simulink model "AZ12"  (R2020a)
settings: Solver=VariableStepAuto  StartTime=0.0  StopTime=6  RelTol=1e-3
libraries: fl_lib x109, ee_lib x35, nesl_utility x16, simulink x3, fl_ps_legacy_lib x1
(part 1 of 2)
settings Model: Creator=sakht system  LastModifiedBy=sakht system

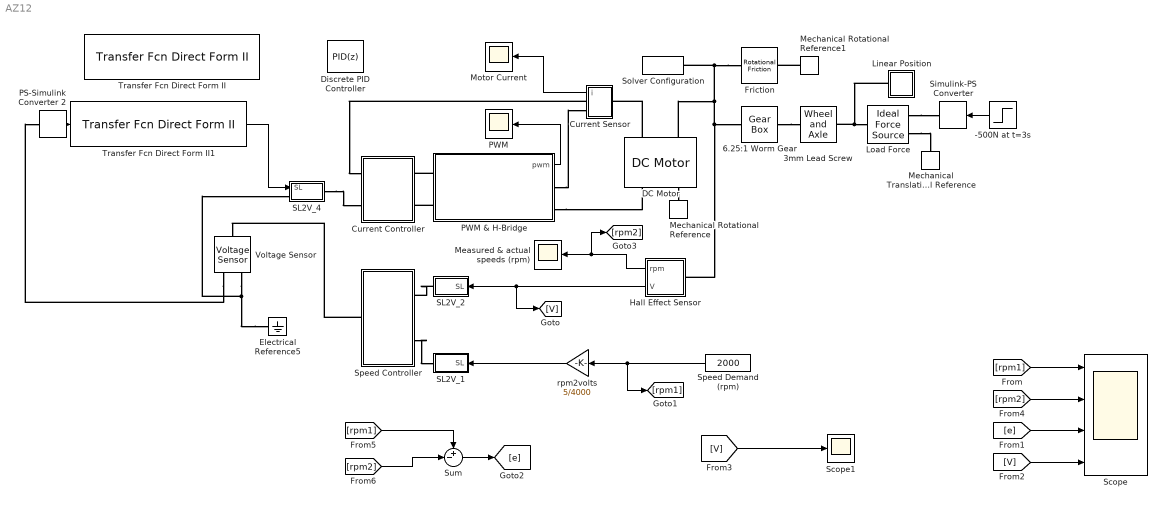
== system AZ12 ==
  -500N at t=3s : Step  Time=3  After=0  SampleTime=0
  3mm Lead Screw : fl_lib/Mechanical/Mechanisms/Wheel and Axle  R=3e-3/(2*pi) m  or=1  t_specify=off  t_priority=High  t=0 N*m  t_nominal_specify=off  t_nominal_unit=N*m  t_nominal_value=1  f_specify=off  f_priority=High  f=0 N  f_nominal_specify=off  f_nominal_unit=N  f_nominal_value=1
  6.25:1 Worm Gear : fl_lib/Mechanical/Mechanisms/Gear Box  ratio=6.25  t_in_specify=off  t_in_priority=High  t_in=0 N*m  t_in_nominal_specify=off  t_in_nominal_unit=N*m  t_in_nominal_value=1  t_out_specify=off  t_out_priority=High  t_out=0 N*m  t_out_nominal_specify=off  t_out_nominal_unit=N*m  t_out_nominal_value=1
  Current Controller : Subsystem
  Current Sensor : Subsystem
  DC Motor : ee_lib/Electromechanical/Brushed Motors/DC Motor  field_option=ee.enum.field_option.pm  Rf=100 Ohm  Lf=1 H  Laf=0.15 H  If0=0 A  parameterization=1  Ra=4.8 Ohm  La=1600e-6 H  emf_or_torque=2  Kv=0.0637 V/rpm  Ki=0.066 N*m/A  T_stall=3e-3*4000/(2*pi*6.25) N*m  w_max=3250 rpm  w_rated=2375 rpm  P_rated=19 W  V_rated=24 V  J=2.5e-5 kg*m^2  lam_param=1  lam=1e-08 N*m/(rad/s)  i_noload=0 A  V_i_noload=1.5 V  speed0=0 rpm  alpha=3.93e-3 1/K  Tmeas=25 degC  thermal_mass=100 J/K  initial_temperature=25 degC
  Discrete PID Controller : simulink/Continuous/PID Controller  Controller=PID  Form=Parallel  TimeDomain=Discrete-time  UseExternalTs=off  SampleTime=0.002  IntegratorMethod=Forward Euler  FilterMethod=Forward Euler  ControllerParametersSource=internal  P=2.4  I=5  D=0.02  UseFilter=on  N=10  TunerSelectOption=Transfer Function Based (PID Tuner App)  InitialConditionSource=internal  InitialConditionForIntegrator=0  InitialConditionForFilter=0  DifferentiatorICPrevScaledInput=0  ExternalReset=none  TrackingMode=off  Kt=1  LimitOutput=off  UpperSaturationLimit=inf  LowerSaturationLimit=-inf  LinearizeAsGain=off  AntiWindupMode=none  Kb=1  POutMin=[]  POutMax=[]  IOutMin=[]  IOutMax=[]  DOutMin=[]  DOutMax=[]  NOutMin=[]  NOutMax=[]  SumOutMin=[]  SumOutMax=[]  SaturationOutMin=[]  SaturationOutMax=[]  PParamMin=[]  PParamMax=[]  IParamMin=[]  IParamMax=[]  DParamMin=[]  DParamMax=[]  NParamMin=[]  NParamMax=[]  KbParamMin=[]  KbParamMax=[]  KtParamMin=[]  KtParamMax=[]  KbOutMin=[]  KbOutMax=[]  KtOutMin=[]  KtOutMax=[]  IntegratorOutMin=[]  IntegratorOutMax=[]  FilterOutMin=[]  FilterOutMax=[]  SumI1OutMin=[]  SumI1OutMax=[]  SumI2OutMin=[]  SumI2OutMax=[]  SumI3OutMin=[]  SumI3OutMax=[]  SumI4OutMin=[]  SumI4OutMax=[]  SumDOutMin=[]  SumDOutMax=[]  DifferentiatorOutMin=[]  DifferentiatorOutMax=[]  FilterDiffOutCoefMin=[]  FilterDiffOutCoefMax=[]  ReciprocalOutMin=[]  ReciprocalOutMax=[]  SumDenOutMin=[]  SumDenOutMax=[]  SumNumOutMin=[]  SumNumOutMax=[]  DivideOutMin=[]  DivideOutMax=[]  UdiffTsProdOutMin=[]  UdiffTsProdOutMax=[]  NTsProdOutMin=[]  NTsProdOutMax=[]  UintegralTsProdOutMin=[]  UintegralTsProdOutMax=[]  UngainTsProdOutMin=[]  UngainTsProdOutMax=[]  IntegratorContinuousStateAttributes=''  IntegratorStateMustResolveToSignalObject=off  IntegratorRTWStateStorageClass=Auto  FilterContinuousStateAttributes=''  FilterStateMustResolveToSignalObject=off  FilterRTWStateStorageClass=Auto  ParallelPVariant=InternalParameters  IdealPVariant=Disabled  IVariant=InternalParameters  DVariant=InternalParameters  IntegratorVariant=Discrete  SatVariant=Disabled  AWVariant=Passthrough  PCopyVariant=Disabled  TRVariant=Disabled  FdbkBlocksVariant=Forward  IdealPFdbkVariant=Disabled  SatFdbkVariant=Disabled  DerivativeFilterVariant=ForwardEulerFilter  NVariant=InternalParameters  NCopyVariant=Disabled  FilterICVariant=InternalICsFilter  IntegratorICVariant=InternalICs  ExternalResetVariant=Disabled  TRSumVariant=Passthrough  SumFdbkVariant=Disabled  SumVariant=Sum_PID  TsampFilterVariant=InternalTs  TsampNgainVariant=Passthrough  TsampIntegralVariant=Passthrough
  Electrical Reference5 : fl_lib/Electrical/Electrical Elements/Electrical Reference
  Friction : fl_lib/Mechanical/Rotational Elements/Rotational Friction  brkwy_trq=0.022 N*m  brkwy_vel=0.03347 rad/s  Col_trq=0.022 N*m  visc_coef=0 N*m/(rad/s)  w_specify=off  w_priority=High  w=0 rad/s  w_nominal_specify=off  w_nominal_unit=rad/s  w_nominal_value=1  t_specify=off  t_priority=High  t=0 N*m  t_nominal_specify=off  t_nominal_unit=N*m  t_nominal_value=1
  Hall Effect Sensor : Subsystem
  Linear Position : Subsystem
  Load Force : fl_lib/Mechanical/Mechanical Sources/Ideal Force Source
  Measured & actual speeds (rpm) : Scope
  Mechanical Rotational Reference : fl_lib/Mechanical/Rotational Elements/Mechanical Rotational Reference
  Mechanical Rotational Reference1 : fl_lib/Mechanical/Rotational Elements/Mechanical Rotational Reference
  Mechanical Translational Reference : fl_lib/Mechanical/Translational Elements/Mechanical Translational Reference
  Motor Current : Scope
  PS-Simulink Converter 2 : nesl_utility/PS-Simulink Converter  PhysicalDomain=network_engine_domain  SubClassName=ps_output  LeftPortType=input  RightPortType=output  PseudoPeriodic=off  Frequencies=[]  Unit=V  AffineConversion=off
  PWM : Scope
  PWM & H-Bridge : Subsystem  Variant=on  VariantControlMode=Label  LabelModeActiveChoice=pwm_choice==1
      settings: AttributesFormatString=%<BlockChoice>
  SL2V_1 : Subsystem
  SL2V_2 : Subsystem
  SL2V_4 : Subsystem
  Scope : Scope  NumInputPorts=4
  Scope1 : Scope
  Simulink-PS Converter : nesl_utility/Simulink-PS Converter  PhysicalDomain=network_engine_domain  SubClassName=ps_input  LeftPortType=input  RightPortType=output  PseudoPeriodic=off  Frequencies=[]  NoiseDistribution=none  NoiseParameters=[]  Unit=N  AffineConversion=off  FilteringAndDerivatives=zero  SimscapeFilterOrder=1  InputFilterTimeConstant=.001  UdotUserProvided=0
  Solver Configuration : nesl_utility/Solver Configuration  PhysicalDomain=network_engine_domain  SubClassName=solver  LeftPortType=input  RightPortType=generic  Tones=[]  Harmonics=[]  SimulateNoise=off  Profile=off  UseLocalSampling=off  EnableSwitchedLinearOptims=on  FrequencyDomain=off  UseCCode=off  RelTol=0.001  AbsTol=1e-06  MinStep=1e-09  ToWorkspace=off  RevertToSquareIcSolve=off  NumHomotopyIterations=100  PhasorMode=off  PhasorModeNumHarmonics=1  DoDC=off  ResidualTolerance=1e-9  UseLocalSolver=off  LocalSolverChoice=NE_BACKWARD_EULER_ADVANCER  LocalSolverSampleTime=.001  DoFixedCost=off  MaxNonlinIter=3  MaxModeIter=2  LinearAlgebra=Sparse  EquationFormulation=NE_TIME_EF  DelaysMemoryBudget=1024  AutomaticFiltering=on  FilteringTimeConstant=0.001  PartitionStorageMethod=AS_NEEDED  PartitionMemoryBudget=1024  PartitionMethod=FAST
  Speed Controller : Subsystem
  Speed Demand (rpm) : Constant  Value=2000
  Sum : Sum  Inputs=+-|
  Transfer Fcn Direct Form II : simulink/Additional Math & Discrete/Additional Discrete/Transfer Fcn Direct Form II  NumCoefVec=[0.31 -0.0034 0]  DenCoefVec=[-0.0058 0]  vinit=0.0  DoSatur=off
      settings: SourceProductBaseCode=SL
  Transfer Fcn Direct Form II1 : simulink/Additional Math & Discrete/Additional Discrete/Transfer Fcn Direct Form II  NumCoefVec=[0.017 -0.0044 0.00340]  DenCoefVec=[0 -0.00077 -0.002]  vinit=0.0  DoSatur=off
      settings: SourceProductBaseCode=SL
  Voltage Sensor : fl_lib/Electrical/Electrical Sensors/Voltage Sensor
  rpm2volts : Gain  Gain=5/4000
  wires:
  [V] -> Scope/4
  [rpm1] -> Scope/1
  Hall Effect Sensor/1(rpm) -> [rpm2], Measured & actual speeds (rpm)/1
  [V] -> Scope1/1
  [rpm2] -> Scope/2
  rpm2volts/1 -> SL2V_1/1(SL)
  [e] -> Scope/3
  Current Sensor/1(i) -> Motor Current/1
  Speed Demand (rpm)/1 -> rpm2volts/1, [rpm1]
  -500N at t=3s/1 -> Simulink-PS Converter/1
  Transfer Fcn Direct Form II1/1 -> SL2V_4/1(SL)
  Hall Effect Sensor/2(V) -> [V], SL2V_2/1(SL)
  PWM & H-Bridge/1(pwm) -> PWM/1
  PS-Simulink Converter 2/1 -> Transfer Fcn Direct Form II1/1
  Sum/1 -> [e]
  [rpm1] -> Sum/1
  [rpm2] -> Sum/2
  connections:
  Friction/LConn1 -- Hall Effect Sensor/LConn1 -- 6.25:1 Worm Gear/LConn1 -- DC Motor/LConn2 -- Solver Configuration/RConn1
  Electrical Reference5/LConn1 -- Voltage Sensor/RConn2 -- SL2V_4/LConn1
  3mm Lead Screw/RConn1 -- Linear Position/LConn1 -- Load Force/LConn1
  Speed Controller/RConn1 -- Voltage Sensor/LConn1
  DC Motor/RConn2 -- Mechanical Rotational Reference/LConn1
  Voltage Sensor/RConn1 -- PS-Simulink Converter 2/LConn1
  Load Force/RConn1 -- Simulink-PS Converter/RConn1
  Speed Controller/LConn2 -- SL2V_1/RConn1
  PWM & H-Bridge/RConn2 -- DC Motor/RConn1
  PWM & H-Bridge/LConn1 -- Current Controller/RConn1
  SL2V_2/RConn1 -- Speed Controller/LConn1
  Current Sensor/RConn1 -- Current Controller/LConn1
  Load Force/RConn2 -- Mechanical Translational Reference/LConn1
  PWM & H-Bridge/RConn1 -- Current Sensor/RConn2
  6.25:1 Worm Gear/RConn1 -- 3mm Lead Screw/LConn1
  PWM & H-Bridge/LConn2 -- Current Controller/RConn2
  DC Motor/LConn1 -- Current Sensor/LConn1
  Mechanical Rotational Reference1/LConn1 -- Friction/RConn1
  SL2V_4/RConn1 -- Current Controller/LConn2

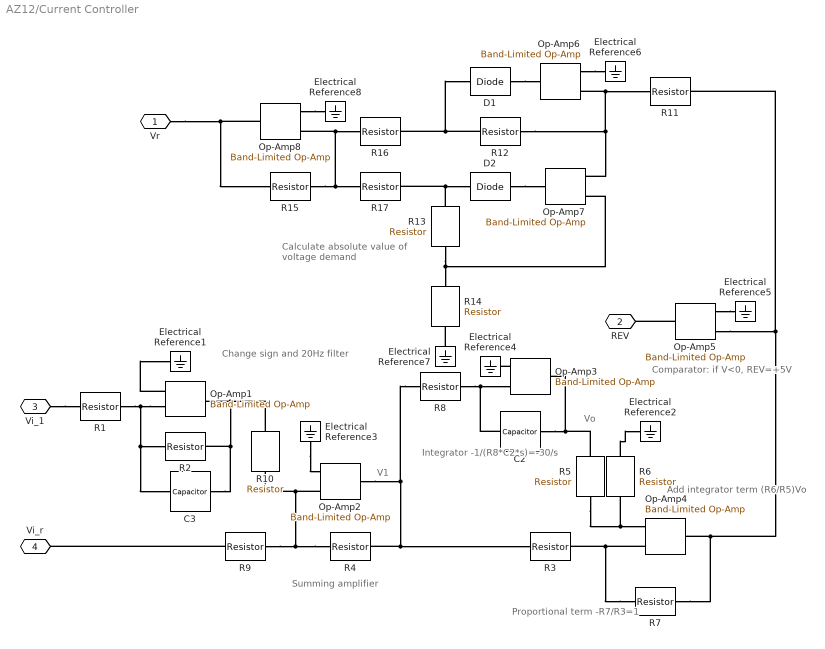
== system AZ12/Current Controller ==
  note: Summing
      | amplifier
  note: Integrator
      | -1/(R8*C2*s)=-30/s
  note: Proportional
      | term -R7/R3=1
  note: Add integrator
      | term (R6/R5)Vo
  note: Vo
  note: V1
  note: Change sign
      | and 20Hz filter
  note: Comparator: if
      | V<0, REV=+5V
  note: Calculate absolute value
      | of voltage demand
  C2 : fl_lib/Electrical/Electrical Elements/Capacitor  c=10 uF  r=0.1 Ohm  g=0 1/Ohm  i_specify=off  i_priority=High  i=0 A  i_nominal_specify=off  i_nominal_unit=A  i_nominal_value=1  v_specify=off  v_priority=High  v=0 V  v_nominal_specify=off  v_nominal_unit=V  v_nominal_value=1  vc_specify=on  vc_priority=High  vc=0 V  vc_nominal_specify=off  vc_nominal_unit=V  vc_nominal_value=1
  C3 : fl_lib/Electrical/Electrical Elements/Capacitor  c=0.8 uF  r=0.1 Ohm  g=0 1/Ohm  i_specify=off  i_priority=High  i=0 A  i_nominal_specify=off  i_nominal_unit=A  i_nominal_value=1  v_specify=off  v_priority=High  v=0 V  v_nominal_specify=off  v_nominal_unit=V  v_nominal_value=1  vc_specify=on  vc_priority=High  vc=0 V  vc_nominal_specify=off  vc_nominal_unit=V  vc_nominal_value=1
  D1 : ee_lib/Semiconductors & Converters/Diode  ModelType=ee.enum.diode.modelType.pwl  Vf=0.6 V  Ron=0.3 Ohm  Goff=1e-08 1/Ohm  prmExp=1  I12="[  0.07 1.5 ] A"  V12="[  0.7 0.8 ] V"  IS=1e-14 A  ec=1  I1=0.0137 A  V1=0.6 V  RS=0 Ohm  Tmeas=298.15 K  N_series=1  N_parallel=1  Rz=0.3 Ohm  BV=inf V  C_param=1  CJ=5 pF  CJ0=50 pF  VJ=1 V  Mgrad=0.5  Vvec="[  0.1 10 100 ] V"  Cvec="[  3.5 1 0.4 ] pF"  FC=0.5  Q_param=ee.enum.diode.recoveryParam.off  iRM=-7.15 A  iF=4 A  didt=-750 A/us  trr_factor=3  trr=115 ns  Qrr=1500 s*uA  TT=50 ns  tau=100 ns  T_param=1  IS_T2=1.25e-7 A  I1_T2=0.245 A  V1_T2=0.5 V  Tmeas2=125 degC  EG_param=1  EG=1.11 eV  XTI_param=1  XTI=3  dBVdT=0 V/K  Tdevice=25 degC  i_specify=off  i_priority=None  i=0 A  i_nominal_specify=off  i_nominal_unit=A  i_nominal_value=1  v_specify=off  v_priority=None  v=0 V  v_nominal_specify=off  v_nominal_unit=V  v_nominal_value=1  i_capacitor_specify=off  i_capacitor_priority=None  i_capacitor=0 A  i_capacitor_nominal_specify=off  i_capacitor_nominal_unit=A  i_capacitor_nominal_value=1  v_capacitor_specify=off  v_capacitor_priority=None  v_capacitor=0 V  v_capacitor_nominal_specify=off  v_capacitor_nominal_unit=V  v_capacitor_nominal_value=1  power_dissipated_specify=off  power_dissipated_priority=None  power_dissipated=0 W  power_dissipated_nominal_specify=off  power_dissipated_nominal_unit=W  power_dissipated_nominal_value=1  thermal_network_parameterization=ee.enum.thermalNetworkTopology.cauer  Rth=[0, 10] K/W  Rth_Foster=[4, 6] K/W  thermal_mass_parameterization=ee.enum.thermalNetwork.timeconstant  thermal_mass=[0, 1] J/K  thermal_mass_Foster=[1.5, 3] J/K  thermal_time_constant=[0, 10] s  thermal_time_constant_Foster=[6, 18] s  thermal_mass_initial_temperatures=[25, 25] degC
  D2 : ee_lib/Semiconductors & Converters/Diode  ModelType=ee.enum.diode.modelType.pwl  Vf=0.6 V  Ron=0.3 Ohm  Goff=1e-08 1/Ohm  prmExp=1  I12="[  0.07 1.5 ] A"  V12="[  0.7 0.8 ] V"  IS=1e-14 A  ec=1  I1=0.0137 A  V1=0.6 V  RS=0 Ohm  Tmeas=298.15 K  N_series=1  N_parallel=1  Rz=0.3 Ohm  BV=inf V  C_param=1  CJ=5 pF  CJ0=50 pF  VJ=1 V  Mgrad=0.5  Vvec="[  0.1 10 100 ] V"  Cvec="[  3.5 1 0.4 ] pF"  FC=0.5  Q_param=ee.enum.diode.recoveryParam.off  iRM=-7.15 A  iF=4 A  didt=-750 A/us  trr_factor=3  trr=115 ns  Qrr=1500 s*uA  TT=50 ns  tau=100 ns  T_param=1  IS_T2=1.25e-7 A  I1_T2=0.245 A  V1_T2=0.5 V  Tmeas2=125 degC  EG_param=1  EG=1.11 eV  XTI_param=1  XTI=3  dBVdT=0 V/K  Tdevice=25 degC  i_specify=off  i_priority=None  i=0 A  i_nominal_specify=off  i_nominal_unit=A  i_nominal_value=1  v_specify=off  v_priority=None  v=0 V  v_nominal_specify=off  v_nominal_unit=V  v_nominal_value=1  i_capacitor_specify=off  i_capacitor_priority=None  i_capacitor=0 A  i_capacitor_nominal_specify=off  i_capacitor_nominal_unit=A  i_capacitor_nominal_value=1  v_capacitor_specify=off  v_capacitor_priority=None  v_capacitor=0 V  v_capacitor_nominal_specify=off  v_capacitor_nominal_unit=V  v_capacitor_nominal_value=1  power_dissipated_specify=off  power_dissipated_priority=None  power_dissipated=0 W  power_dissipated_nominal_specify=off  power_dissipated_nominal_unit=W  power_dissipated_nominal_value=1  thermal_network_parameterization=ee.enum.thermalNetworkTopology.cauer  Rth=[0, 10] K/W  Rth_Foster=[4, 6] K/W  thermal_mass_parameterization=ee.enum.thermalNetwork.timeconstant  thermal_mass=[0, 1] J/K  thermal_mass_Foster=[1.5, 3] J/K  thermal_time_constant=[0, 10] s  thermal_time_constant_Foster=[6, 18] s  thermal_mass_initial_temperatures=[25, 25] degC
  Electrical Reference{1..8} (8 alike) : fl_lib/Electrical/Electrical Elements/Electrical Reference
  Op-Amp{1..8} (8 alike) : ee_lib/Integrated Circuits/Band-Limited Op-Amp  A=1000  Rin=1e+06 Ohm  Rout=100 Ohm  Vmin=-5 V  Vmax=5 V  Vdotmax=1000 V/s  f=1e3 Hz  V0=0 V
      settings: SourceProductBaseCode=PS
  R{1..7,9..17} (16 alike) : fl_lib/Electrical/Electrical Elements/Resistor  R=10 kOhm  i_specify=off  i_priority=High  i=0 A  i_nominal_specify=off  i_nominal_unit=A  i_nominal_value=1  v_specify=off  v_priority=High  v=0 V  v_nominal_specify=off  v_nominal_unit=V  v_nominal_value=1
  R8 : fl_lib/Electrical/Electrical Elements/Resistor  R=3.3 kOhm  i_specify=off  i_priority=High  i=0 A  i_nominal_specify=off  i_nominal_unit=A  i_nominal_value=1  v_specify=off  v_priority=High  v=0 V  v_nominal_specify=off  v_nominal_unit=V  v_nominal_value=1
  Vr : PMIOPort  Side=Right
  REV : PMIOPort  Port=2  Side=Right
  Vi_1 : PMIOPort  Port=3  Side=Left
  Vi_r : PMIOPort  Port=4  Side=Left
  connections:
  R9/LConn1 -- Vi_r/RConn1
  R8/LConn1 -- Op-Amp2/RConn1 -- R3/LConn1 -- R4/RConn1
  R8/RConn1 -- Op-Amp3/LConn2 -- C2/LConn1
  R5/LConn1 -- Op-Amp3/RConn1 -- C2/RConn1
  Op-Amp5/LConn2 -- R11/RConn1 -- R7/RConn1 -- Op-Amp4/RConn1
  R6/LConn1 -- Op-Amp4/LConn1 -- R5/RConn1
  R7/LConn1 -- Op-Amp4/LConn2 -- R3/RConn1
  R4/LConn1 -- Op-Amp2/LConn2 -- R10/RConn1 -- R9/RConn1
  Op-Amp1/LConn2 -- R2/LConn1 -- C3/LConn1 -- R1/RConn1
  Op-Amp1/RConn1 -- R2/RConn1 -- C3/RConn1 -- R10/LConn1
  Op-Amp1/LConn1 -- Electrical Reference1/LConn1
  Op-Amp3/LConn1 -- Electrical Reference4/LConn1
  Electrical Reference3/LConn1 -- Op-Amp2/LConn1
  R6/RConn1 -- Electrical Reference2/LConn1
  Vi_1/RConn1 -- R1/LConn1
  Op-Amp5/LConn1 -- Electrical Reference5/LConn1
  Op-Amp5/RConn1 -- REV/RConn1
  R12/RConn1 -- Op-Amp6/LConn2 -- R11/LConn1 -- Op-Amp7/LConn1
  Op-Amp6/LConn1 -- Electrical Reference6/LConn1
  R13/RConn1 -- R14/LConn1 -- Op-Amp7/LConn2
  Electrical Reference7/LConn1 -- R14/RConn1
  D1/RConn1 -- Op-Amp6/RConn1
  R12/LConn1 -- D1/LConn1 -- R16/RConn1
  D2/RConn1 -- Op-Amp7/RConn1
  R13/LConn1 -- D2/LConn1 -- R17/RConn1
  Vr/RConn1 -- Op-Amp8/RConn1 -- R15/LConn1
  R15/RConn1 -- Op-Amp8/LConn2 -- R16/LConn1 -- R17/LConn1
  Op-Amp8/LConn1 -- Electrical Reference8/LConn1

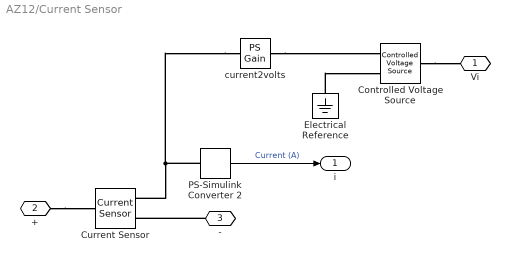
== system AZ12/Current Sensor ==
  Controlled Voltage Source : fl_lib/Electrical/Electrical Sources/Controlled Voltage Source
  Current Sensor : fl_lib/Electrical/Electrical Sensors/Current Sensor
  Electrical Reference : fl_lib/Electrical/Electrical Elements/Electrical Reference
  PS-Simulink Converter 2 : nesl_utility/PS-Simulink Converter  PhysicalDomain=network_engine_domain  SubClassName=ps_output  LeftPortType=input  RightPortType=output  PseudoPeriodic=off  Frequencies=[]  Unit=A  AffineConversion=off
  current2volts : fl_ps_legacy_lib/Legacy Physical Signals/Functions/PS Gain  gain=1
  Vi : PMIOPort  Side=Right
  + : PMIOPort  Port=2  Side=Right
  - : PMIOPort  Port=3  Side=Left
  i : Outport
  wires:
  PS-Simulink Converter 2/1 -> i/1  "Current (A)"
  connections:
  +/RConn1 -- Current Sensor/LConn1
  -/RConn1 -- Current Sensor/RConn2
  current2volts/LConn1 -- PS-Simulink Converter 2/LConn1 -- Current Sensor/RConn1
  Electrical Reference/LConn1 -- Controlled Voltage Source/RConn2
  Controlled Voltage Source/LConn1 -- Vi/RConn1
  current2volts/RConn1 -- Controlled Voltage Source/RConn1

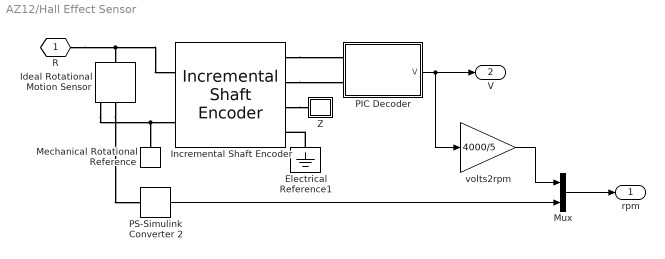
== system AZ12/Hall Effect Sensor ==
  Electrical Reference1 : fl_lib/Electrical/Electrical Elements/Electrical Reference
  Ideal Rotational Motion Sensor : fl_lib/Mechanical/Mechanical Sensors/Ideal Rotational Motion Sensor  wrap_angle=simscape.enum.onoff.off  offset=0 rad
  Incremental Shaft Encoder : ee_lib/Sensors & Transducers/Incremental Shaft Encoder  NPulse=2  Vm=5 V  angle0=0 deg
      settings: SourceProductBaseCode=PS  InternalSimscapePortConfiguration="{\"Bottom\":[],\"Left\":[{\"id\":\"R\",\"label\":\"R\",\"type\":\"foundation.mechanical.rotational.rotational\"},{\"id\":\"C\",\"label\":\"C\",\"type\":\"foundation.mechanical.rotational.rotational\"}],\"Right\":[{\"id\":\"A\",\"label\":\"A\",\"type\":\"foundation.electrical.electrical\"},{\"id\":\"B\",\"label\":\"B\",\"type\":\"foundation.electrical.electrical\"},{\"id\":\"Z\",\"label\":\"Z\",\"type\":\"foundation.electrical.electrical\"},{\"id\":\"GND\",\"label\":\"REF\",\"type\":\"foundation.electrical.electrical\"}],\"Top\":[]}"
  Mechanical Rotational Reference : fl_lib/Mechanical/Rotational Elements/Mechanical Rotational Reference
  Mux : Mux  Inputs=2
  PIC Decoder : Subsystem
  PS-Simulink Converter 2 : nesl_utility/PS-Simulink Converter  PhysicalDomain=network_engine_domain  SubClassName=ps_output  LeftPortType=input  RightPortType=output  PseudoPeriodic=off  Frequencies=[]  Unit=rpm  AffineConversion=off
  Z : Subsystem
  volts2rpm : Gain  Gain=4000/5
  R : PMIOPort  Side=Left
  rpm : Outport
  V : Outport  Port=2
  wires:
  PS-Simulink Converter 2/1 -> Mux/2
  Mux/1 -> rpm/1
  PIC Decoder/1(V) -> volts2rpm/1, V/1
  volts2rpm/1 -> Mux/1
  connections:
  Ideal Rotational Motion Sensor/RConn2 -- PS-Simulink Converter 2/LConn1
  Ideal Rotational Motion Sensor/RConn1 -- Incremental Shaft Encoder/LConn2 -- Mechanical Rotational Reference/LConn1
  R/RConn1 -- Ideal Rotational Motion Sensor/LConn1 -- Incremental Shaft Encoder/LConn1
  Electrical Reference1/LConn1 -- Incremental Shaft Encoder/RConn4
  Incremental Shaft Encoder/RConn3 -- Z/LConn1
  Incremental Shaft Encoder/RConn1 -- PIC Decoder/LConn1
  Incremental Shaft Encoder/RConn2 -- PIC Decoder/LConn2

== system AZ12/Linear Position ==
  Linear Position (mm) : Scope
  Linear Speed (mm/s) : Scope
  Mechanical Translational Reference : fl_lib/Mechanical/Translational Elements/Mechanical Translational Reference
  PS-Simulink Converter 1 : nesl_utility/PS-Simulink Converter  PhysicalDomain=network_engine_domain  SubClassName=ps_output  LeftPortType=input  RightPortType=output  PseudoPeriodic=off  Frequencies=[]  Unit=mm/s  AffineConversion=off
  PS-Simulink Converter 3 : nesl_utility/PS-Simulink Converter  PhysicalDomain=network_engine_domain  SubClassName=ps_output  LeftPortType=input  RightPortType=output  PseudoPeriodic=off  Frequencies=[]  Unit=mm  AffineConversion=off
  Sensor1 : fl_lib/Mechanical/Mechanical Sensors/Ideal Translational Motion Sensor  offset=0 m
  P : PMIOPort  Side=Left
  wires:
  PS-Simulink Converter 3/1 -> Linear Position (mm)/1
  PS-Simulink Converter 1/1 -> Linear Speed (mm/s)/1
  connections:
  Sensor1/RConn1 -- Mechanical Translational Reference/LConn1
  Sensor1/RConn3 -- PS-Simulink Converter 3/LConn1
  P/RConn1 -- Sensor1/LConn1
  Sensor1/RConn2 -- PS-Simulink Converter 1/LConn1

== system AZ12/PWM & H-Bridge ==
  Implementation : Subsystem  VariantControl=pwm_choice==3
  System-Averaged : Subsystem  VariantControl=pwm_choice==1
  System-PWM : Subsystem  VariantControl=pwm_choice==2
  Vr : PMIOPort  Side=Left
  REV : PMIOPort  Port=2  Side=Left
  V+ : PMIOPort  Port=3  Side=Right
  V- : PMIOPort  Port=4  Side=Right
  pwm : Outport

== system AZ12/SL2V_1 ==
  SL : Inport
  Controlled Voltage Source : fl_lib/Electrical/Electrical Sources/Controlled Voltage Source
  Electrical Reference : fl_lib/Electrical/Electrical Elements/Electrical Reference
  Simulink-PS Converter : nesl_utility/Simulink-PS Converter  PhysicalDomain=network_engine_domain  SubClassName=ps_input  LeftPortType=input  RightPortType=output  PseudoPeriodic=off  Frequencies=[]  NoiseDistribution=none  NoiseParameters=[]  Unit=V  AffineConversion=off  FilteringAndDerivatives=zero  SimscapeFilterOrder=1  InputFilterTimeConstant=.001  UdotUserProvided=0
  V : PMIOPort  Side=Right
  wires:
  SL/1 -> Simulink-PS Converter/1
  connections:
  Electrical Reference/LConn1 -- Controlled Voltage Source/RConn2
  V/RConn1 -- Controlled Voltage Source/LConn1
  Simulink-PS Converter/RConn1 -- Controlled Voltage Source/RConn1

== system AZ12/SL2V_2 ==
  SL : Inport
  Controlled Voltage Source : fl_lib/Electrical/Electrical Sources/Controlled Voltage Source
  Electrical Reference : fl_lib/Electrical/Electrical Elements/Electrical Reference
  Simulink-PS Converter : nesl_utility/Simulink-PS Converter  PhysicalDomain=network_engine_domain  SubClassName=ps_input  LeftPortType=input  RightPortType=output  PseudoPeriodic=off  Frequencies=[]  NoiseDistribution=none  NoiseParameters=[]  Unit=V  AffineConversion=off  FilteringAndDerivatives=zero  SimscapeFilterOrder=1  InputFilterTimeConstant=.001  UdotUserProvided=0
  V : PMIOPort  Side=Right
  wires:
  SL/1 -> Simulink-PS Converter/1
  connections:
  Simulink-PS Converter/RConn1 -- Controlled Voltage Source/RConn1
  V/RConn1 -- Controlled Voltage Source/LConn1
  Electrical Reference/LConn1 -- Controlled Voltage Source/RConn2

== system AZ12/SL2V_4 ==
  SL : Inport
  Controlled Voltage Source : fl_lib/Electrical/Electrical Sources/Controlled Voltage Source
  Electrical Reference : fl_lib/Electrical/Electrical Elements/Electrical Reference
  Simulink-PS Converter : nesl_utility/Simulink-PS Converter  PhysicalDomain=network_engine_domain  SubClassName=ps_input  LeftPortType=input  RightPortType=output  PseudoPeriodic=off  Frequencies=[]  NoiseDistribution=none  NoiseParameters=[]  Unit=V  AffineConversion=off  FilteringAndDerivatives=zero  SimscapeFilterOrder=1  InputFilterTimeConstant=.001  UdotUserProvided=0
  V : PMIOPort  Side=Right
  V1 : PMIOPort  Port=2  Side=Left
  wires:
  SL/1 -> Simulink-PS Converter/1
  connections:
  Electrical Reference/LConn1 -- V1/RConn1 -- Controlled Voltage Source/RConn2
  V/RConn1 -- Controlled Voltage Source/LConn1
  Simulink-PS Converter/RConn1 -- Controlled Voltage Source/RConn1

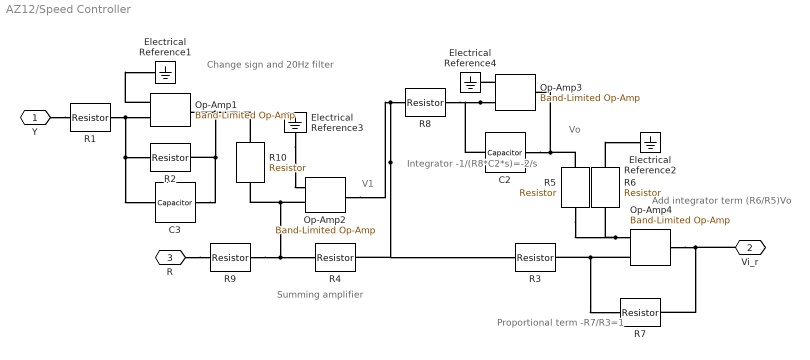
== system AZ12/Speed Controller ==
  note: Summing
      | amplifier
  note: Integrator
      | -1/(R8*C2*s)=-2/s
  note: Proportional
      | term -R7/R3=1
  note: Add integrator
      | term (R6/R5)Vo
  note: Vo
  note: V1
  note: Change sign
      | and 20Hz filter
  C2 : fl_lib/Electrical/Electrical Elements/Capacitor  c=10 uF  r=0.1 Ohm  g=0 1/Ohm  i_specify=off  i_priority=High  i=0 A  i_nominal_specify=off  i_nominal_unit=A  i_nominal_value=1  v_specify=off  v_priority=High  v=0 V  v_nominal_specify=off  v_nominal_unit=V  v_nominal_value=1  vc_specify=on  vc_priority=High  vc=0 V  vc_nominal_specify=off  vc_nominal_unit=V  vc_nominal_value=1
  C3 : fl_lib/Electrical/Electrical Elements/Capacitor  c=0.8 uF  r=0.1 Ohm  g=0 1/Ohm  i_specify=off  i_priority=High  i=0 A  i_nominal_specify=off  i_nominal_unit=A  i_nominal_value=1  v_specify=off  v_priority=High  v=0 V  v_nominal_specify=off  v_nominal_unit=V  v_nominal_value=1  vc_specify=on  vc_priority=High  vc=0 V  vc_nominal_specify=off  vc_nominal_unit=V  vc_nominal_value=1
  Electrical Reference{1..4} (4 alike) : fl_lib/Electrical/Electrical Elements/Electrical Reference
  Op-Amp{1..4} (4 alike) : ee_lib/Integrated Circuits/Band-Limited Op-Amp  A=1000  Rin=1e+06 Ohm  Rout=100 Ohm  Vmin=-5 V  Vmax=5 V  Vdotmax=1000 V/s  f=1e3 Hz  V0=0 V
      settings: SourceProductBaseCode=PS
  R{1..7,9..10} (9 alike) : fl_lib/Electrical/Electrical Elements/Resistor  R=10 kOhm  i_specify=off  i_priority=High  i=0 A  i_nominal_specify=off  i_nominal_unit=A  i_nominal_value=1  v_specify=off  v_priority=High  v=0 V  v_nominal_specify=off  v_nominal_unit=V  v_nominal_value=1
  R8 : fl_lib/Electrical/Electrical Elements/Resistor  R=55 kOhm  i_specify=off  i_priority=High  i=0 A  i_nominal_specify=off  i_nominal_unit=A  i_nominal_value=1  v_specify=off  v_priority=High  v=0 V  v_nominal_specify=off  v_nominal_unit=V  v_nominal_value=1
  Y : PMIOPort  Side=Left
  Vi_r : PMIOPort  Port=2  Side=Right
  R : PMIOPort  Port=3  Side=Left
  connections:
  R8/LConn1 -- Op-Amp2/RConn1 -- R4/RConn1 -- R3/LConn1
  Op-Amp3/LConn2 -- R8/RConn1 -- C2/LConn1
  R5/LConn1 -- Op-Amp3/RConn1 -- C2/RConn1
  Op-Amp4/RConn1 -- Vi_r/RConn1 -- R7/RConn1
  Op-Amp4/LConn1 -- R6/LConn1 -- R5/RConn1
  Op-Amp4/LConn2 -- R7/LConn1 -- R3/RConn1
  Op-Amp2/LConn2 -- R10/RConn1 -- R4/LConn1 -- R9/RConn1
  R1/RConn1 -- Op-Amp1/LConn2 -- C3/LConn1 -- R2/LConn1
  R10/LConn1 -- Op-Amp1/RConn1 -- C3/RConn1 -- R2/RConn1
  Y/RConn1 -- R1/LConn1
  Electrical Reference3/LConn1 -- Op-Amp2/LConn1
  Op-Amp1/LConn1 -- Electrical Reference1/LConn1
  R/RConn1 -- R9/LConn1
  R6/RConn1 -- Electrical Reference2/LConn1
  Op-Amp3/LConn1 -- Electrical Reference4/LConn1

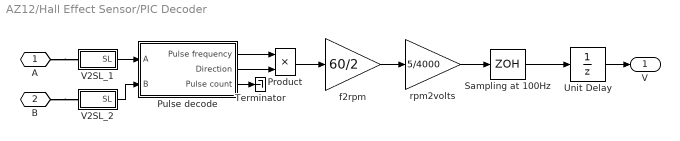
== system AZ12/Hall Effect Sensor/PIC Decoder ==
  Product : Product  RndMeth=Zero
  Pulse decode : Subsystem
  Sampling at 100Hz : ZeroOrderHold  SampleTime=0.01
  Terminator : Terminator
  Unit Delay : UnitDelay  SampleTime=0.01  HasFrameUpgradeWarning=on
  V2SL_1 : Subsystem
  V2SL_2 : Subsystem
  f2rpm : Gain  Gain=60/2
  rpm2volts : Gain  Gain=5/4000
  A : PMIOPort  Side=Left
  B : PMIOPort  Port=2  Side=Left
  V : Outport
  wires:
  Product/1 -> f2rpm/1
  Pulse decode/2(Direction) -> Product/2
  Pulse decode/1(Pulse frequency) -> Product/1
  Pulse decode/3(Pulse count) -> Terminator/1
  f2rpm/1 -> rpm2volts/1
  rpm2volts/1 -> Sampling at 100Hz/1
  V2SL_1/1(SL) -> Pulse decode/1(A)
  V2SL_2/1(SL) -> Pulse decode/2(B)
  Sampling at 100Hz/1 -> Unit Delay/1
  Unit Delay/1 -> V/1
  connections:
  A/RConn1 -- V2SL_1/LConn1
  B/RConn1 -- V2SL_2/LConn1

== system AZ12/Hall Effect Sensor/Z ==
  Electrical Reference1 : fl_lib/Electrical/Electrical Elements/Electrical Reference
  PS-Simulink Converter 2 : nesl_utility/PS-Simulink Converter  PhysicalDomain=network_engine_domain  SubClassName=ps_output  LeftPortType=input  RightPortType=output  PseudoPeriodic=off  Frequencies=[]  Unit=V  AffineConversion=off
  Voltage Sensor : fl_lib/Electrical/Electrical Sensors/Voltage Sensor
  Vz : Scope
  u : PMIOPort  Side=Left
  wires:
  PS-Simulink Converter 2/1 -> Vz/1
  connections:
  Voltage Sensor/RConn2 -- Electrical Reference1/LConn1
  Voltage Sensor/RConn1 -- PS-Simulink Converter 2/LConn1
  u/RConn1 -- Voltage Sensor/LConn1

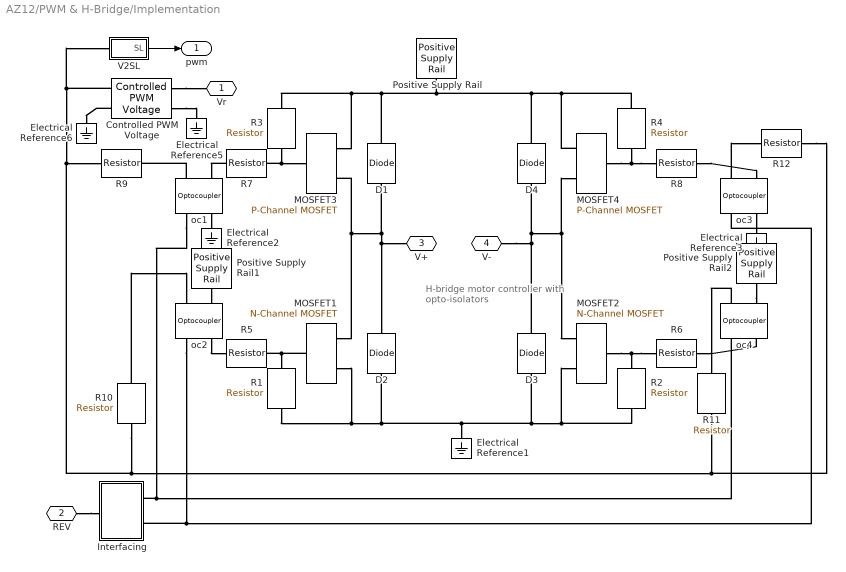
== system AZ12/PWM & H-Bridge/Implementation ==
  note: H-bridge motor
      | controller with
      | opto-isolators
  Controlled PWM Voltage : ee_lib/Integrated Circuits/Controlled PWM Voltage  F=10000 Hz  TD=0 s  pulse_width_offset=0 s  pulse_min=0 s  Vmin=0 V  Vmax=5 V  Vm=5 V  pwm_or_av=1  event_type=1  sample_time=1e-6 s  u_min=0  u_max=1
  D{1..4} (4 alike) : fl_lib/Electrical/Electrical Elements/Diode  Vf=0.6 V  Ron=0.3 Ohm  Goff=1e-08 1/Ohm  i_specify=off  i_priority=High  i=0 A  i_nominal_specify=off  i_nominal_unit=A  i_nominal_value=1  v_specify=off  v_priority=High  v=0 V  v_nominal_specify=off  v_nominal_unit=V  v_nominal_value=1
  Electrical Reference{1..3,5..6} (5 alike) : fl_lib/Electrical/Electrical Elements/Electrical Reference
  Interfacing : Subsystem
  MOSFET1 : ee_lib/Semiconductors & Converters/N-Channel MOSFET  paramTerminal=ee.enum.mosfet.numberOfTerminals.three  parameterization=2  prmDatasheet=1  prmEquCoeff=1  Beta=5 A/V^2  Rds=0.025 Ohm  Id=6 A  Vgs=10 V  Vth=5 V  Vth0=1.7 V  lam=0 1/V  gamma_vth=0.5 V^0.50000  phib=0.5 V  Vth1=1.9071 V  Vbs1=-1 V  Vth2=2.066 V  Vbs2=-2 V  Tmeas=25 degC  RS=0.001 Ohm  RD=0.001 Ohm  RB=0.001 Ohm  C_param=1  C_GS=270 pF  C_GD=80 pF  C_DS=0 pF  C_iss=350 pF  C_rss=80 pF  C_oss=0 pF  charge_linearity_param=1  C_OX=200 pF  V_C_OX=-0.5 V  C_iss_vec=[ 720 700 590 470 390 310 ] pF  C_rss_vec=[ 450 400 300 190 95 55 ] pF  C_oss_vec=[ 900 810 690 420 270 170 ] pF  C_GS_vec=[ 270 300 290 280 295 255 ] pF  C_GD_vec=[ 450 400 300 190 95 55 ] pF  C_DS_vec=[ 450 410 390 230 175 115 ] pF  C_Vds_vec=[ 0.1 0.3 1 3 10 30 ] V  V_GS_for_cap_data=NaN V  charge_linearity_param_vgb=ee.enum.mosfet.cgbLinearity.instantly  IsDiode=0 A  Vbi=0.6 V  n=1  Cj0Diode=0 pF  TT=50e-9 s  dVth_dT=-6 mV/K  dVth0_dT=-6 mV/K  Rds_T2=0.037 Ohm  Tmeas2=125 degC  BEXDatasheet=-1.5  BEXEquCoeff=-1.5  etaisDatasheet=3  etaisEquCoeff=3  TdeviceDatasheet=25 degC  TdeviceEquCoeff=25 degC  thermal_network_parameterization=ee.enum.thermalNetworkTopology.cauer  Rth=[0, 10] K/W  Rth_Foster=[4, 6] K/W  thermal_mass_parameterization=ee.enum.thermalNetwork.timeconstant  thermal_mass=[0, 1] J/K  thermal_mass_Foster=[1.5, 3] J/K  thermal_time_constant=[0, 10] s  thermal_time_constant_Foster=[6, 18] s  thermal_mass_initial_temperatures=[25, 25] degC  betaref=18 A/V^2  Vfbref=-1.1 V  gamma=3.5 V^0.50000  phib2ref=1 V  thesatref=0.4 1/V  alpha=0  Vp=5e-2 V  thesrref=0 1/V  m=8  Tref=25 degC  Cox=1500 pF  Cgso=100 pF  Cgdo=14 pF  Rsref=2e-3 Ohm  Rdref=0.17 Ohm  Rgref=8.4 Ohm  Rbref=2e-3 Ohm  Isref=5.2e-13 A  Cj0=480 pF  Tprm=1  etabet=1.3  Stvfb=5e-4 V/K  Stphib=-8.5e-4 V/K  etasat=1.04  etasr=0.65  etar=0.95  etais=3  Tsim=25 degC  T0=[25, 25] degC
  MOSFET2 : ee_lib/Semiconductors & Converters/N-Channel MOSFET  paramTerminal=ee.enum.mosfet.numberOfTerminals.three  parameterization=2  prmDatasheet=1  prmEquCoeff=1  Beta=5 A/V^2  Rds=0.025 Ohm  Id=6 A  Vgs=10 V  Vth=5 V  Vth0=1.7 V  lam=0 1/V  gamma_vth=0.5 V^0.50000  phib=0.5 V  Vth1=1.9071 V  Vbs1=-1 V  Vth2=2.066 V  Vbs2=-2 V  Tmeas=25 degC  RS=0.001 Ohm  RD=0.001 Ohm  RB=0.001 Ohm  C_param=1  C_GS=270 pF  C_GD=80 pF  C_DS=0 pF  C_iss=350 pF  C_rss=80 pF  C_oss=0 pF  charge_linearity_param=1  C_OX=200 pF  V_C_OX=-0.5 V  C_iss_vec=[ 720 700 590 470 390 310 ] pF  C_rss_vec=[ 450 400 300 190 95 55 ] pF  C_oss_vec=[ 900 810 690 420 270 170 ] pF  C_GS_vec=[ 270 300 290 280 295 255 ] pF  C_GD_vec=[ 450 400 300 190 95 55 ] pF  C_DS_vec=[ 450 410 390 230 175 115 ] pF  C_Vds_vec=[ 0.1 0.3 1 3 10 30 ] V  V_GS_for_cap_data=NaN V  charge_linearity_param_vgb=ee.enum.mosfet.cgbLinearity.instantly  IsDiode=0 A  Vbi=0.6 V  n=1  Cj0Diode=0 pF  TT=50e-9 s  dVth_dT=-6 mV/K  dVth0_dT=-6 mV/K  Rds_T2=0.037 Ohm  Tmeas2=125 degC  BEXDatasheet=-1.5  BEXEquCoeff=-1.5  etaisDatasheet=3  etaisEquCoeff=3  TdeviceDatasheet=25 degC  TdeviceEquCoeff=25 degC  thermal_network_parameterization=ee.enum.thermalNetworkTopology.cauer  Rth=[0, 10] K/W  Rth_Foster=[4, 6] K/W  thermal_mass_parameterization=ee.enum.thermalNetwork.timeconstant  thermal_mass=[0, 1] J/K  thermal_mass_Foster=[1.5, 3] J/K  thermal_time_constant=[0, 10] s  thermal_time_constant_Foster=[6, 18] s  thermal_mass_initial_temperatures=[25, 25] degC  betaref=18 A/V^2  Vfbref=-1.1 V  gamma=3.5 V^0.50000  phib2ref=1 V  thesatref=0.4 1/V  alpha=0  Vp=5e-2 V  thesrref=0 1/V  m=8  Tref=25 degC  Cox=1500 pF  Cgso=100 pF  Cgdo=14 pF  Rsref=2e-3 Ohm  Rdref=0.17 Ohm  Rgref=8.4 Ohm  Rbref=2e-3 Ohm  Isref=5.2e-13 A  Cj0=480 pF  Tprm=1  etabet=1.3  Stvfb=5e-4 V/K  Stphib=-8.5e-4 V/K  etasat=1.04  etasr=0.65  etar=0.95  etais=3  Tsim=25 degC  T0=[25, 25] degC
  MOSFET3 : ee_lib/Semiconductors & Converters/P-Channel MOSFET  paramTerminal=ee.enum.mosfet.numberOfTerminals.three  parameterization=2  prmDatasheet=1  prmEquCoeff=1  Beta=2 A/V^2  Rds=0.04 Ohm  Id=-6 A  Vgs=-10 V  Vth=-5 V  Vth0=-1.4 V  lam=0 1/V  gamma_vth=0.5 V^0.50000  phib=0.5 V  Vth1=-1.6071 V  Vbs1=1 V  Vth2=-1.7660 V  Vbs2=2 V  Tmeas=25 degC  RS=0.001 Ohm  RD=0.001 Ohm  RB=0.001 Ohm  C_param=1  C_GS=225 pF  C_GD=45 pF  C_DS=0 pF  C_iss=270 pF  C_rss=45 pF  C_oss=0 pF  charge_linearity_param=1  C_OX=200 pF  V_C_OX=0.5 V  C_iss_vec=[ 225 215 200 190 180 170 ] pF  C_rss_vec=[ 75 60 50 35 25 20 ] pF  C_oss_vec=[ 180 160 125 80 60 45 ] pF  C_GS_vec=[ 150 150 150 150 150 150 ] pF  C_GD_vec=[ 75 60 50 35 25 20 ] pF  C_DS_vec=[ 105 100 75 45 35 25 ] pF  C_Vsd_vec=[ 0.1 0.3 1 3 10 30 ] V  V_GS_for_cap_data=NaN V  charge_linearity_param_vgb=ee.enum.mosfet.cgbLinearity.instantly  IsDiode=0 A  Vbi=0.6 V  n=1  Cj0Diode=0 pF  TT=50e-9 s  dVth_dT=2 mV/K  dVth0_dT=2 mV/K  Rds_T2=0.25 Ohm  Tmeas2=125 degC  BEXDatasheet=-1.5  BEXEquCoeff=-1.5  etaisDatasheet=3  etaisEquCoeff=3  TdeviceDatasheet=25 degC  TdeviceEquCoeff=25 degC  thermal_network_parameterization=ee.enum.thermalNetworkTopology.cauer  Rth=[0, 10] K/W  Rth_Foster=[4, 6] K/W  thermal_mass_parameterization=ee.enum.thermalNetwork.timeconstant  thermal_mass=[0, 1] J/K  thermal_mass_Foster=[1.5, 3] J/K  thermal_time_constant=[0, 10] s  thermal_time_constant_Foster=[6, 18] s  thermal_mass_initial_temperatures=[25, 25] degC  betaref=18 A/V^2  Vfbref=-1.1 V  gamma=3.5 V^0.50000  phib2ref=1 V  thesatref=0.4 1/V  alpha=0  Vp=5e-2 V  thesrref=0 1/V  m=8  Tref=25 degC  Cox=1500 pF  Cgso=100 pF  Cgdo=14 pF  Rsref=2e-3 Ohm  Rdref=0.17 Ohm  Rgref=8.4 Ohm  Rbref=2e-3 Ohm  Isref=5.2e-13 A  Cj0=480 pF  Tprm=1  etabet=1.3  Stvfb=5e-4 V/K  Stphib=-8.5e-4 V/K  etasat=1.04  etasr=0.65  etar=0.95  etais=3  Tsim=25 degC  T0=[25, 25] degC
      settings: SourceProductBaseCode=PS  InternalSimscapePortConfiguration="{\"Bottom\":[],\"Left\":[{\"id\":\"G\",\"label\":\"\",\"type\":\"foundation.electrical.electrical\"}],\"Right\":[{\"id\":\"S\",\"label\":\"s\",\"type\":\"foundation.electrical.electrical\"},{\"id\":\"D\",\"label\":\"d\",\"type\":\"foundation.electrical.electrical\"}],\"Top\":[]}"
  MOSFET4 : ee_lib/Semiconductors & Converters/P-Channel MOSFET  paramTerminal=ee.enum.mosfet.numberOfTerminals.three  parameterization=2  prmDatasheet=1  prmEquCoeff=1  Beta=2 A/V^2  Rds=0.04 Ohm  Id=-6 A  Vgs=-10 V  Vth=-5 V  Vth0=-1.4 V  lam=0 1/V  gamma_vth=0.5 V^0.50000  phib=0.5 V  Vth1=-1.6071 V  Vbs1=1 V  Vth2=-1.7660 V  Vbs2=2 V  Tmeas=25 degC  RS=0.001 Ohm  RD=0.001 Ohm  RB=0.001 Ohm  C_param=1  C_GS=225 pF  C_GD=45 pF  C_DS=0 pF  C_iss=270 pF  C_rss=45 pF  C_oss=0 pF  charge_linearity_param=1  C_OX=200 pF  V_C_OX=0.5 V  C_iss_vec=[ 225 215 200 190 180 170 ] pF  C_rss_vec=[ 75 60 50 35 25 20 ] pF  C_oss_vec=[ 180 160 125 80 60 45 ] pF  C_GS_vec=[ 150 150 150 150 150 150 ] pF  C_GD_vec=[ 75 60 50 35 25 20 ] pF  C_DS_vec=[ 105 100 75 45 35 25 ] pF  C_Vsd_vec=[ 0.1 0.3 1 3 10 30 ] V  V_GS_for_cap_data=NaN V  charge_linearity_param_vgb=ee.enum.mosfet.cgbLinearity.instantly  IsDiode=0 A  Vbi=0.6 V  n=1  Cj0Diode=0 pF  TT=50e-9 s  dVth_dT=2 mV/K  dVth0_dT=2 mV/K  Rds_T2=0.25 Ohm  Tmeas2=125 degC  BEXDatasheet=-1.5  BEXEquCoeff=-1.5  etaisDatasheet=3  etaisEquCoeff=3  TdeviceDatasheet=25 degC  TdeviceEquCoeff=25 degC  thermal_network_parameterization=ee.enum.thermalNetworkTopology.cauer  Rth=[0, 10] K/W  Rth_Foster=[4, 6] K/W  thermal_mass_parameterization=ee.enum.thermalNetwork.timeconstant  thermal_mass=[0, 1] J/K  thermal_mass_Foster=[1.5, 3] J/K  thermal_time_constant=[0, 10] s  thermal_time_constant_Foster=[6, 18] s  thermal_mass_initial_temperatures=[25, 25] degC  betaref=18 A/V^2  Vfbref=-1.1 V  gamma=3.5 V^0.50000  phib2ref=1 V  thesatref=0.4 1/V  alpha=0  Vp=5e-2 V  thesrref=0 1/V  m=8  Tref=25 degC  Cox=1500 pF  Cgso=100 pF  Cgdo=14 pF  Rsref=2e-3 Ohm  Rdref=0.17 Ohm  Rgref=8.4 Ohm  Rbref=2e-3 Ohm  Isref=5.2e-13 A  Cj0=480 pF  Tprm=1  etabet=1.3  Stvfb=5e-4 V/K  Stphib=-8.5e-4 V/K  etasat=1.04  etasr=0.65  etar=0.95  etais=3  Tsim=25 degC  T0=[25, 25] degC
      settings: SourceProductBaseCode=PS  InternalSimscapePortConfiguration="{\"Bottom\":[],\"Left\":[{\"id\":\"G\",\"label\":\"\",\"type\":\"foundation.electrical.electrical\"}],\"Right\":[{\"id\":\"S\",\"label\":\"s\",\"type\":\"foundation.electrical.electrical\"},{\"id\":\"D\",\"label\":\"d\",\"type\":\"foundation.electrical.electrical\"}],\"Top\":[]}"
  Positive Supply Rail : ee_lib/Sources/Positive Supply Rail  v0=24 V
      settings: SourceProductBaseCode=PS  InternalSimscapePortConfiguration="{\"Bottom\":[],\"Left\":[],\"Right\":[{\"id\":\"p\",\"label\":\"\",\"type\":\"foundation.electrical.electrical\"}],\"Top\":[]}"
  Positive Supply Rail1 : ee_lib/Sources/Positive Supply Rail  v0=24 V
      settings: SourceProductBaseCode=PS  InternalSimscapePortConfiguration="{\"Bottom\":[],\"Left\":[],\"Right\":[{\"id\":\"p\",\"label\":\"\",\"type\":\"foundation.electrical.electrical\"}],\"Top\":[]}"
  Positive Supply Rail2 : ee_lib/Sources/Positive Supply Rail  v0=24 V
      settings: SourceProductBaseCode=PS  InternalSimscapePortConfiguration="{\"Bottom\":[],\"Left\":[],\"Right\":[{\"id\":\"p\",\"label\":\"\",\"type\":\"foundation.electrical.electrical\"}],\"Top\":[]}"
  R{1..4} (4 alike) : fl_lib/Electrical/Electrical Elements/Resistor  R=10e3 Ohm  i_specify=off  i_priority=High  i=0 A  i_nominal_specify=off  i_nominal_unit=A  i_nominal_value=1  v_specify=off  v_priority=High  v=0 V  v_nominal_specify=off  v_nominal_unit=V  v_nominal_value=1
  R{9..12} (4 alike) : fl_lib/Electrical/Electrical Elements/Resistor  R=470 Ohm  i_specify=off  i_priority=High  i=0 A  i_nominal_specify=off  i_nominal_unit=A  i_nominal_value=1  v_specify=off  v_priority=High  v=0 V  v_nominal_specify=off  v_nominal_unit=V  v_nominal_value=1
  R{5..8} (4 alike) : fl_lib/Electrical/Electrical Elements/Resistor  R=1e3 Ohm  i_specify=off  i_priority=High  i=0 A  i_nominal_specify=off  i_nominal_unit=A  i_nominal_value=1  v_specify=off  v_priority=High  v=0 V  v_nominal_specify=off  v_nominal_unit=V  v_nominal_value=1
  V2SL : Subsystem
  oc{1..4} (4 alike) : ee_lib/Semiconductors & Converters/Optocoupler  CTR=0.2  prmExp=1  I12="[  0.001 0.015 ] A"  V12="[  0.9 1.05 ] V"  IS=1e-10 A  ec=2  RS=0 Ohm  Tmeas=298.15 K  C_param=1  CJ=50 pF  CJ0=50 pF  VJ=1 V  Mgrad=0.5  Vvec="[  0.1 10 100 ] V"  Cvec="[  3.5 1 0.4 ] pF"  FC=0.5  T_param=1  IS_T2=1.8e-8 A  I1_T2=0.029 A  V1_T2=1.05 V  Tmeas2=125 degC  EG_param=1  EG=1.11 eV  XTI_param=1  XTI=3  Tdevice=25 degC  i_capacitor_specify=off  i_capacitor_priority=High  i_capacitor=0 A  i_capacitor_nominal_specify=off  i_capacitor_nominal_unit=A  i_capacitor_nominal_value=1  v_capacitor_specify=off  v_capacitor_priority=None  v_capacitor=0 V  v_capacitor_nominal_specify=off  v_capacitor_nominal_unit=V  v_capacitor_nominal_value=1  thermal_network_parameterization=ee.enum.thermalNetworkTopology.cauer  Rth=[0, 10] K/W  Rth_Foster=[4, 6] K/W  thermal_mass_parameterization=ee.enum.thermalNetwork.timeconstant  thermal_mass=[0, 1] J/K  thermal_mass_Foster=[1.5, 3] J/K  thermal_time_constant=[0, 10] s  thermal_time_constant_Foster=[6, 18] s  thermal_mass_initial_temperatures=[25, 25] degC
      settings: SourceProductBaseCode=PS  InternalSimscapePortConfiguration="{\"Bottom\":[],\"Left\":[{\"id\":\"p\",\"label\":\"\",\"type\":\"foundation.electrical.electrical\"},{\"id\":\"C\",\"label\":\"\",\"type\":\"foundation.electrical.electrical\"}],\"Right\":[{\"id\":\"n\",\"label\":\"\",\"type\":\"foundation.electrical.electrical\"},{\"id\":\"E\",\"label\":\"\",\"type\":\"foundation.electrical.electrical\"}],\"Top\":[]}"
  Vr : PMIOPort  Side=Left
  REV : PMIOPort  Port=2  Side=Left
  V+ : PMIOPort  Port=3  Side=Right
  V- : PMIOPort  Port=4  Side=Right
  pwm : Outport
  wires:
  V2SL/1(SL) -> pwm/1
  connections:
  REV/RConn1 -- Interfacing/LConn1
  Interfacing/RConn2 -- oc3/RConn1 -- oc2/RConn1
  R10/RConn1 -- R11/RConn1 -- R12/RConn1 -- Controlled PWM Voltage/RConn1 -- V2SL/LConn1 -- R9/LConn1
  Interfacing/RConn1 -- oc4/RConn1 -- oc1/RConn1
  R8/RConn1 -- MOSFET4/LConn1 -- R4/RConn1
  Positive Supply Rail/RConn1 -- R3/LConn1 -- MOSFET3/RConn1 -- D1/RConn1 -- MOSFET4/RConn1 -- R4/LConn1 -- D4/RConn1
  R3/RConn1 -- MOSFET3/LConn1 -- R7/RConn1
  R6/RConn1 -- MOSFET2/LConn1 -- R2/LConn1
  R5/RConn1 -- MOSFET1/LConn1 -- R1/LConn1
  R2/RConn1 -- MOSFET2/RConn2 -- D3/LConn1 -- D2/LConn1 -- MOSFET1/RConn2 -- R1/RConn1 -- Electrical Reference1/LConn1
  D4/LConn1 -- D3/RConn1 -- V-/RConn1 -- MOSFET4/RConn2 -- MOSFET2/RConn1
  D1/LConn1 -- MOSFET1/RConn1 -- MOSFET3/RConn2 -- V+/RConn1 -- D2/RConn1
  oc1/LConn1 -- R9/RConn1
  R6/LConn1 -- oc4/RConn2
  oc3/RConn2 -- Electrical Reference3/LConn1
  R7/LConn1 -- oc1/LConn2
  Positive Supply Rail1/RConn1 -- oc2/LConn2
  oc1/RConn2 -- Electrical Reference2/LConn1
  Positive Supply Rail2/RConn1 -- oc4/LConn2
  oc4/LConn1 -- R11/LConn1
  Controlled PWM Voltage/LConn1 -- Vr/RConn1
  oc3/LConn1 -- R12/LConn1
  Controlled PWM Voltage/LConn2 -- Electrical Reference5/LConn1
  oc2/RConn2 -- R5/LConn1
  R8/LConn1 -- oc3/LConn2
  R10/LConn1 -- oc2/LConn1
  Controlled PWM Voltage/RConn2 -- Electrical Reference6/LConn1

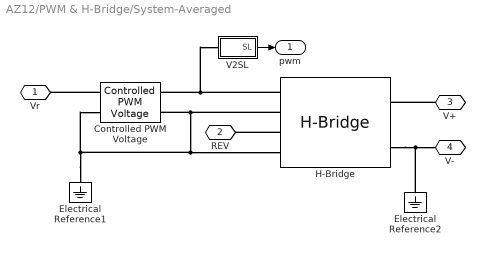
== system AZ12/PWM & H-Bridge/System-Averaged ==
  Controlled PWM Voltage : ee_lib/Integrated Circuits/Controlled PWM Voltage  F=10000 Hz  TD=0 s  pulse_width_offset=0 s  pulse_min=0 s  Vmin=0 V  Vmax=5 V  Vm=5 V  pwm_or_av=2  event_type=1  sample_time=1e-6 s  u_min=0  u_max=1
  Electrical Reference1 : fl_lib/Electrical/Electrical Elements/Electrical Reference
  Electrical Reference2 : fl_lib/Electrical/Electrical Elements/Electrical Reference
  H-Bridge : ee_lib/Semiconductors & Converters/Converters/H-Bridge  supply_ports=ee.enum.supply_ports.hidesupply  Venable=2.5 V  Vmax=5 V  Vreverse=2.5 V  Vbrake=2.5 V  Vm=24 V  pwm_or_av=2  regenerative_braking_mode=2  discontinuous=0  freewheeling_mode=1  Ron=0.1 Ohm  Don=0.1 Ohm  Goff=1e-6 S  Rload=10 Ohm  Lload=1e-5 H  F=10 kHz  thermal_mass=100 J/K  initial_temperature=298.15 K  Ron2=0.1 Ohm  Don2=0.05 Ohm  Tmeas=298.15 K  Tmeas2=398.15 K
  V2SL : Subsystem
  Vr : PMIOPort  Side=Left
  REV : PMIOPort  Port=2  Side=Left
  V+ : PMIOPort  Port=3  Side=Right
  V- : PMIOPort  Port=4  Side=Right
  pwm : Outport
  wires:
  V2SL/1(SL) -> pwm/1
  connections:
  V+/RConn1 -- H-Bridge/RConn1
  H-Bridge/RConn2 -- Electrical Reference2/LConn1 -- V-/RConn1
  Controlled PWM Voltage/RConn1 -- V2SL/LConn1 -- H-Bridge/LConn1
  Electrical Reference1/LConn1 -- H-Bridge/LConn4 -- H-Bridge/LConn2 -- Controlled PWM Voltage/RConn2 -- Controlled PWM Voltage/LConn2
  Controlled PWM Voltage/LConn1 -- Vr/RConn1
  H-Bridge/LConn3 -- REV/RConn1

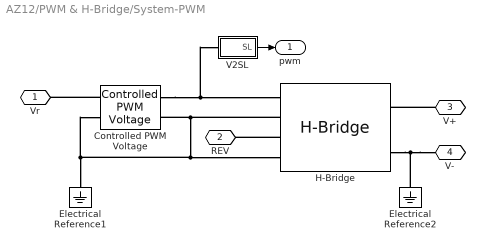
== system AZ12/PWM & H-Bridge/System-PWM ==
  Controlled PWM Voltage : ee_lib/Integrated Circuits/Controlled PWM Voltage  F=10000 Hz  TD=0 s  pulse_width_offset=0 s  pulse_min=0 s  Vmin=0 V  Vmax=5 V  Vm=5 V  pwm_or_av=1  event_type=1  sample_time=1e-6 s  u_min=0  u_max=1
  Electrical Reference1 : fl_lib/Electrical/Electrical Elements/Electrical Reference
  Electrical Reference2 : fl_lib/Electrical/Electrical Elements/Electrical Reference
  H-Bridge : ee_lib/Semiconductors & Converters/Converters/H-Bridge  supply_ports=ee.enum.supply_ports.hidesupply  Venable=2.5 V  Vmax=5 V  Vreverse=2.5 V  Vbrake=2.5 V  Vm=24 V  pwm_or_av=1  regenerative_braking_mode=2  discontinuous=0  freewheeling_mode=1  Ron=0.1 Ohm  Don=0.1 Ohm  Goff=1e-6 S  Rload=10 Ohm  Lload=1e-5 H  F=10 kHz  thermal_mass=100 J/K  initial_temperature=298.15 K  Ron2=0.1 Ohm  Don2=0.05 Ohm  Tmeas=298.15 K  Tmeas2=398.15 K
  V2SL : Subsystem
  Vr : PMIOPort  Side=Left
  REV : PMIOPort  Port=2  Side=Left
  V+ : PMIOPort  Port=3  Side=Right
  V- : PMIOPort  Port=4  Side=Right
  pwm : Outport
  wires:
  V2SL/1(SL) -> pwm/1
  connections:
  H-Bridge/LConn3 -- REV/RConn1
  Controlled PWM Voltage/LConn1 -- Vr/RConn1
  Controlled PWM Voltage/RConn2 -- H-Bridge/LConn2 -- H-Bridge/LConn4 -- Controlled PWM Voltage/LConn2 -- Electrical Reference1/LConn1
  Controlled PWM Voltage/RConn1 -- V2SL/LConn1 -- H-Bridge/LConn1
  V-/RConn1 -- Electrical Reference2/LConn1 -- H-Bridge/RConn2
  V+/RConn1 -- H-Bridge/RConn1

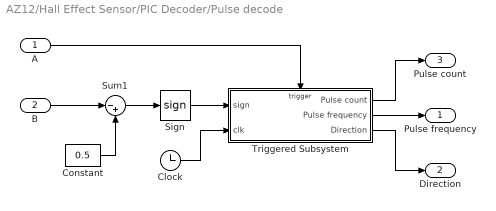
== system AZ12/Hall Effect Sensor/PIC Decoder/Pulse decode ==
  A : Inport
  B : Inport  Port=2
  Clock : Clock
  Constant : Constant  Value=0.5
  Sign : Signum
  Sum1 : Sum  Inputs=|-+
  Triggered Subsystem : Subsystem  TreatAsAtomicUnit=on
  Pulse frequency : Outport
  Direction : Outport  Port=2
  Pulse count : Outport  Port=3
  wires:
  Triggered Subsystem/3(Direction) -> Direction/1
  Triggered Subsystem/2(Pulse frequency) -> Pulse frequency/1
  Clock/1 -> Triggered Subsystem/2(clk)
  Triggered Subsystem/1(Pulse count) -> Pulse count/1
  A/1 -> Triggered Subsystem/Trigger
  Sign/1 -> Triggered Subsystem/1(sign)
  B/1 -> Sum1/1
  Sum1/1 -> Sign/1
  Constant/1 -> Sum1/2

== system AZ12/Hall Effect Sensor/PIC Decoder/V2SL_1 ==
  Electrical Reference1 : fl_lib/Electrical/Electrical Elements/Electrical Reference
  PS-Simulink Converter 2 : nesl_utility/PS-Simulink Converter  PhysicalDomain=network_engine_domain  SubClassName=ps_output  LeftPortType=input  RightPortType=output  PseudoPeriodic=off  Frequencies=[]  Unit=V  AffineConversion=off
  V2logic : Gain  Gain=0.2
  Voltage Sensor : fl_lib/Electrical/Electrical Sensors/Voltage Sensor
  V : PMIOPort  Side=Left
  SL : Outport
  wires:
  PS-Simulink Converter 2/1 -> V2logic/1
  V2logic/1 -> SL/1
  connections:
  Voltage Sensor/RConn2 -- Electrical Reference1/LConn1
  V/RConn1 -- Voltage Sensor/LConn1
  Voltage Sensor/RConn1 -- PS-Simulink Converter 2/LConn1

== system AZ12/Hall Effect Sensor/PIC Decoder/V2SL_2 ==
  Electrical Reference1 : fl_lib/Electrical/Electrical Elements/Electrical Reference
  PS-Simulink Converter 2 : nesl_utility/PS-Simulink Converter  PhysicalDomain=network_engine_domain  SubClassName=ps_output  LeftPortType=input  RightPortType=output  PseudoPeriodic=off  Frequencies=[]  Unit=V  AffineConversion=off
  V2logic : Gain  Gain=0.2
  Voltage Sensor : fl_lib/Electrical/Electrical Sensors/Voltage Sensor
  V : PMIOPort  Side=Left
  SL : Outport
  wires:
  V2logic/1 -> SL/1
  PS-Simulink Converter 2/1 -> V2logic/1
  connections:
  Voltage Sensor/RConn1 -- PS-Simulink Converter 2/LConn1
  V/RConn1 -- Voltage Sensor/LConn1
  Voltage Sensor/RConn2 -- Electrical Reference1/LConn1
